simulink model "blockdiagrams_v2"  (R2022a)
settings: Solver=VariableStepAuto  StartTime=0.0  StopTime=10.0  RelTol=1e-3
settings Model: Creator=tedbrekken  LastModifiedBy=tedbrekken

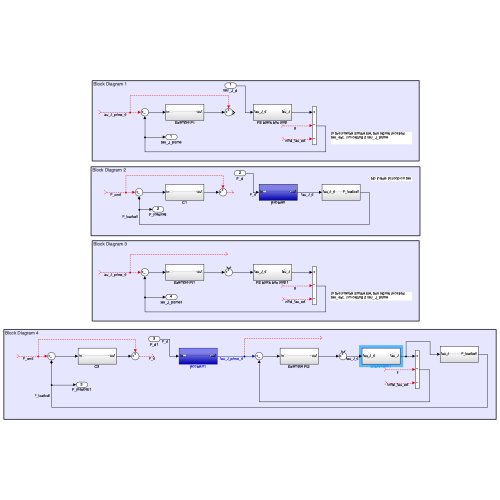
[thumbnail: Simulink's stored preview of the top-level diagram]
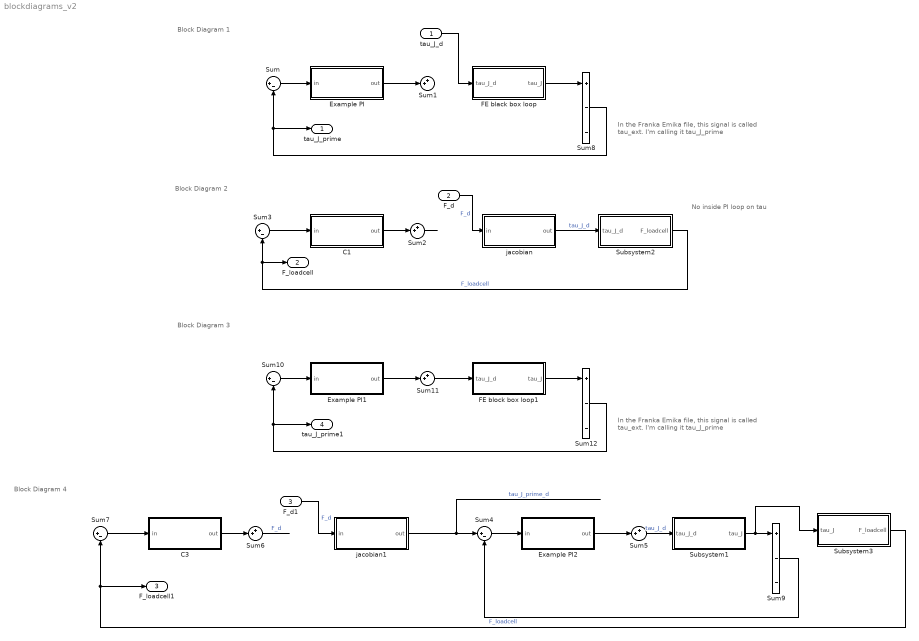
== system blockdiagrams_v2 ==
  note: No inside PI loop on tau
  note: Block Diagram 4
  note: Block Diagram 2
  note: Block Diagram 1
  note: In the Franka Emika file, this signal is called tau_ext. I'm calling it tau_J_prime
  note: In the Franka Emika file, this signal is called tau_ext. I'm calling it tau_J_prime
  note: Block Diagram 3
  tau_J_d : Inport
  F_d : Inport  Port=2
  F_d1 : Inport  Port=3
  C1 : Subsystem
  C3 : Subsystem
  Example PI : Subsystem
  Example PI1 : Subsystem
  Example PI2 : Subsystem
  FE black box loop : Subsystem
  FE block box loop1 : Subsystem
  Subsystem1 : Subsystem
  Subsystem2 : Subsystem
  Subsystem3 : Subsystem
  Sum{,3..4,7,10} (5 alike) : Sum  Inputs=|+-
  Sum{1..2,5..6,11} (5 alike) : Sum  Inputs=++|
  Sum12 : Sum  Inputs=+--
  Sum8 : Sum  Inputs=+--
  Sum9 : Sum  Inputs=+--
  jacobian : Subsystem
  jacobian1 : Subsystem
  tau_J_prime : Outport
  F_loadcell : Outport  Port=2
  F_loadcell1 : Outport  Port=3
  tau_J_prime1 : Outport  Port=4
  wires:
  Sum/1 -> Example PI/1(in)
  Example PI/1(out) -> Sum1/2
  ? -> Sum1/1, Sum/1  "tau_J_prime_d"
  C1/1(out) -> Sum2/2
  jacobian/1(out) -> Subsystem2/1(tau_J_d)  "tau_J_d"
  Sum2/1 -> ?
  Sum3/1 -> C1/1(in)
  ? -> Sum2/1, Sum3/1  "F_cmd"
  Subsystem2/1(F_loadcell) -> F_loadcell/1, Sum3/2  "F_loadcell"
  Sum4/1 -> Example PI2/1(in)
  Sum5/1 -> Subsystem1/1(tau_J_d)  "tau_J_d"
  Example PI2/1(out) -> Sum5/2
  Sum6/1 -> ?  "F_d"
  jacobian1/1(out) -> Sum4/1  "tau_J_prime_d"
  Sum9/1 -> Sum4/2
  Sum7/1 -> C3/1(in)
  ? -> Sum6/1, Sum7/1  "F_cmd"
  C3/1(out) -> Sum6/2
  Subsystem3/1(F_loadcell) -> F_loadcell1/1, Sum7/2  "F_loadcell"
  FE black box loop/1(tau_J) -> Sum8/1
  ? -> Sum8/2  "g"
  ? -> Sum8/3  "initial_tau_ext"
  Sum8/1 -> tau_J_prime/1, Sum/2
  tau_J_d/1 -> FE black box loop/1(tau_J_d)
  F_d/1 -> jacobian/1(in)  "F_d"
  Subsystem1/1(tau_J) -> Subsystem3/1(tau_J), Sum9/1
  ? -> Sum9/3  "initial_tau_ext"
  ? -> Sum9/2  "g"
  F_d1/1 -> jacobian1/1(in)  "F_d"
  ? -> Sum12/3  "initial_tau_ext"
  Sum12/1 -> tau_J_prime1/1, Sum10/2
  Sum10/1 -> Example PI1/1(in)
  ? -> Sum12/2  "g"
  FE block box loop1/1(tau_J) -> Sum12/1
  Example PI1/1(out) -> Sum11/2
  ? -> Sum10/1  "tau_J_prime_d"
  Sum11/1 -> FE block box loop1/1(tau_J_d)

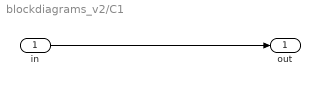
== system blockdiagrams_v2/C1 ==
  in : Inport
  out : Outport
  wires:
  in/1 -> out/1

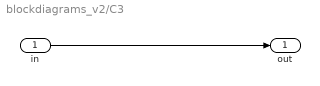
== system blockdiagrams_v2/C3 ==
  in : Inport
  out : Outport
  wires:
  in/1 -> out/1

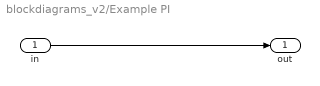
== system blockdiagrams_v2/Example PI ==
  in : Inport
  out : Outport
  wires:
  in/1 -> out/1

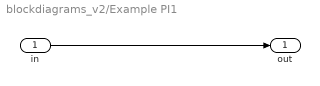
== system blockdiagrams_v2/Example PI1 ==
  in : Inport
  out : Outport
  wires:
  in/1 -> out/1

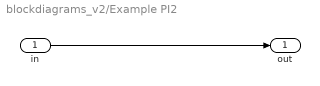
== system blockdiagrams_v2/Example PI2 ==
  in : Inport
  out : Outport
  wires:
  in/1 -> out/1

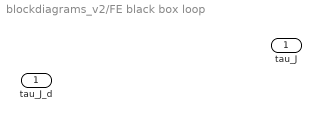
== system blockdiagrams_v2/FE black box loop ==
  tau_J_d : Inport
  tau_J : Outport

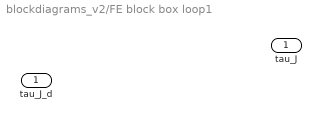
== system blockdiagrams_v2/FE block box loop1 ==
  tau_J_d : Inport
  tau_J : Outport

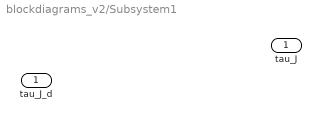
== system blockdiagrams_v2/Subsystem1 ==
  tau_J_d : Inport
  tau_J : Outport

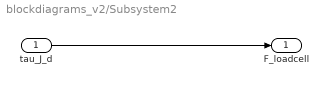
== system blockdiagrams_v2/Subsystem2 ==
  tau_J_d : Inport
  F_loadcell : Outport
  wires:
  tau_J_d/1 -> F_loadcell/1

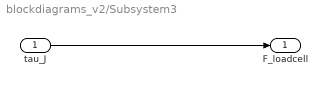
== system blockdiagrams_v2/Subsystem3 ==
  tau_J : Inport
  F_loadcell : Outport
  wires:
  tau_J/1 -> F_loadcell/1

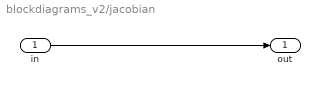
== system blockdiagrams_v2/jacobian ==
  in : Inport
  out : Outport
  wires:
  in/1 -> out/1

== system blockdiagrams_v2/jacobian1 ==
  in : Inport
  out : Outport
  wires:
  in/1 -> out/1
